simulink model "pendulum_sim_model"  (R2023b)
settings: Solver=VariableStepAuto  StartTime=0.0  StopTime=40  MaxStep=0.0001  RelTol=1e-3
values from neighbouring files (symbols this model uses):
  a = 0.1    [pendulum_experiment.m]
  alpha_0 = cutData(1)    [model_validation_data.m]    (also in pendulum_experiment.m)
  Bp_ = 1.46e-5    (= 1.46e-05)    [model_validation_data.m]    (also in pendulum_experiment.m)
  c = 0.1    [pendulum_experiment.m]
  g_ = 9.81    [model_validation_data.m]    (also in pendulum_experiment.m)
  Jp_ = 2.4573e-5    (= 2.4573e-05)    [model_validation_data.m]    (also in pendulum_experiment.m)
  lp_ = Lp/2    (= 0.0645)    [model_validation_data.m]    (also in pendulum_experiment.m)
  mp_ = 0.024    [model_validation_data.m]    (also in pendulum_experiment.m)
libraries: simulink x1
settings Model: Creator=renzo  LastModifiedBy=renzo

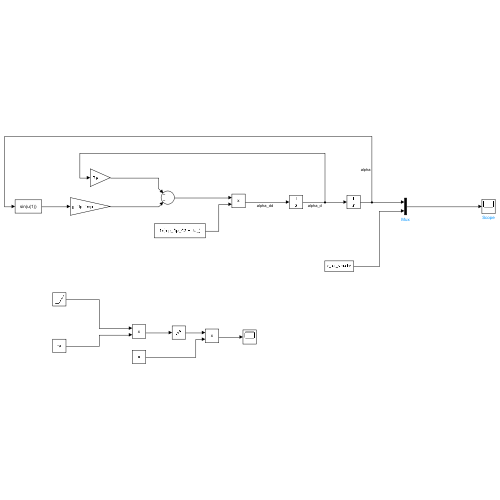
[thumbnail: Simulink's stored preview of the top-level diagram]
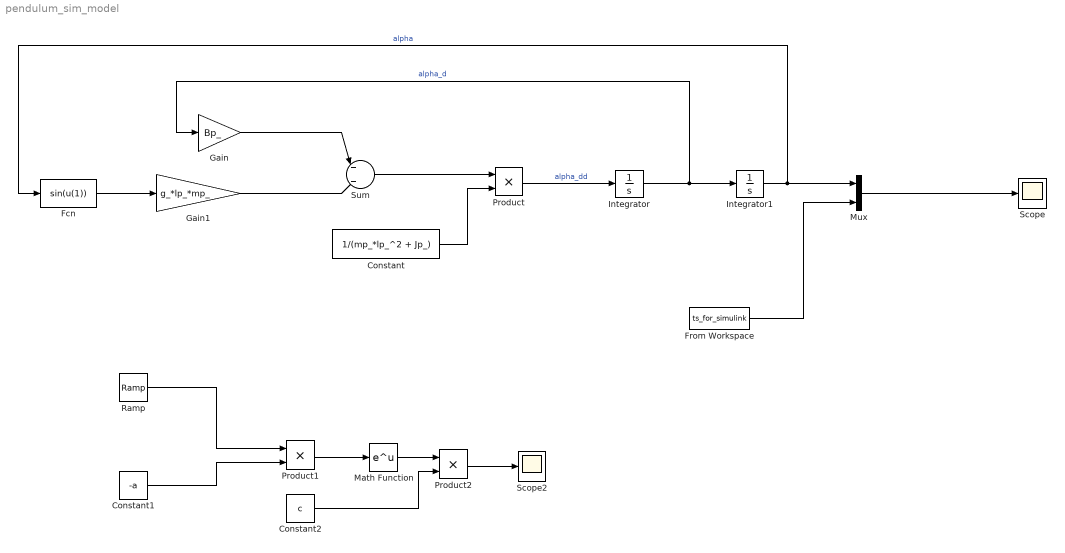
== system pendulum_sim_model ==
  Constant : Constant  Value=1/(mp_*lp_^2 + Jp_)
  Constant1 : Constant  Value=-a
  Constant2 : Constant  Value=c
  Fcn : Fcn  Expr=sin(u(1))
  From Workspace : FromWorkspace  VariableName=ts_for_simulink
  Gain : Gain  Gain=Bp_
  Gain1 : Gain  Gain=g_*lp_*mp_
  Integrator : Integrator
  Integrator1 : Integrator  InitialCondition=alpha_0
  Math Function : Math
  Mux : Mux  Inputs=2
  Product : Product
  Product1 : Product
  Product2 : Product
  Ramp : simulink/Sources/Ramp  slope=1  start=0  InitialOutput=0
  Scope : Scope
  Scope2 : Scope
  Sum : Sum  Inputs=|-|-|
  wires:
  Constant1/1 -> Product1/2
  Math Function/1 -> Product2/1
  Product1/1 -> Math Function/1
  Constant2/1 -> Product2/2
  Product2/1 -> Scope2/1
  Sum/1 -> Product/1
  Constant/1 -> Product/2
  Gain/1 -> Sum/1
  Integrator/1 -> Gain/1, Integrator1/1  "alpha_d"
  Product/1 -> Integrator/1  "alpha_dd"
  Ramp/1 -> Product1/1
  Integrator1/1 -> Fcn/1, Mux/1  "alpha"
  Fcn/1 -> Gain1/1
  Gain1/1 -> Sum/2
  Mux/1 -> Scope/1
  From Workspace/1 -> Mux/2
